simulink model "Standalone_PV_with_MPPT"  (R2024a)
settings: Solver=VariableStepAuto  StartTime=0.0  StopTime=10.0  RelTol=1e-3
libraries: spsSeriesRLCBranchLib x4, spsCurrentMeasurementLib x3, spsMeanLib x2, spsVoltageMeasurementLib x2, spsDiodeLib x1, spsGroundLib x1, spsIGBTLib x1, simulink x1, spsPVArrayLib x1, sps_lib x1
settings Model: Creator=91889  LastModifiedBy=91889

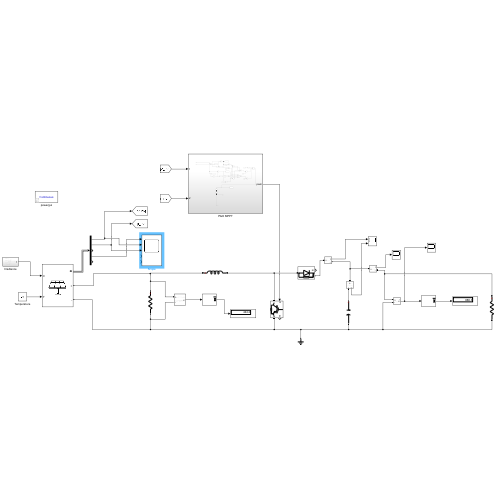
[thumbnail: Simulink's stored preview of the top-level diagram]
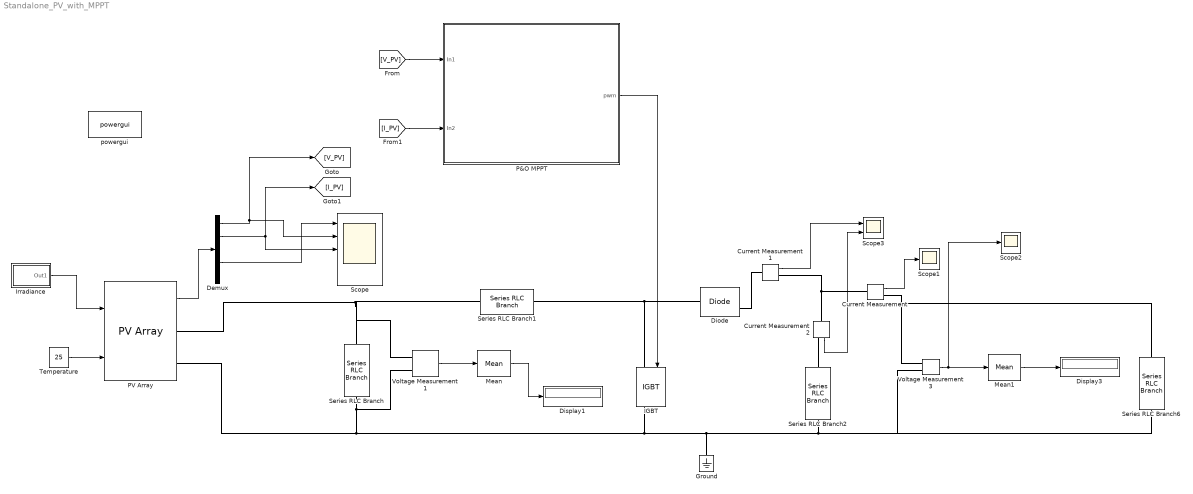
== system Standalone_PV_with_MPPT ==
  Current Measurement : spsCurrentMeasurementLib/Current Measurement  PhasorSimulation=off  OutputType=Complex  PSBequivalent=0
  Current Measurement1 : spsCurrentMeasurementLib/Current Measurement  PhasorSimulation=off  OutputType=Complex  PSBequivalent=0
  Current Measurement2 : spsCurrentMeasurementLib/Current Measurement  PhasorSimulation=off  OutputType=Complex  PSBequivalent=0
  Demux : Demux  Outputs=5
  Diode : spsDiodeLib/Diode  Ron=0.001  Lon=0  Vf=0.8  IC=0  UseSnubber=0  Rs=500  Cs=250e-9  Measurements=on
  Display1 : Display
  Display3 : Display
  Ground : spsGroundLib/Ground  LConnTagsString=a
  IGBT : spsIGBTLib/IGBT  Ron=0.001  Lon=0  Vf=1  Tf=1e-6  Tt=2e-6  IC=0  Rs=1e5  Cs=inf  Measurements=on
  Irradiance : Subsystem
  Mean : spsMeanLib/Mean  Freq=60  Vinit=0  Ts=0
  Mean1 : spsMeanLib/Mean  Freq=60  Vinit=0  Ts=0
  P&O MPPT : Subsystem
  PV Array : spsPVArrayLib/PV Array  Npar=3  Nser=20  PlotType=array @ 1000 W/m2 & specified temperatures  S_vec="[ 1000  500  100 ]"  Temp_C_vec="[ 45 25  ]"  ModuleName=User-defined  PlotWhenSelected=off  Pm=213.15  Ncell=60  Voc=35  Isc=7.84  Vm=29  Im=7.35  beta_Voc_pc=-0.36099  alpha_Isc_pc=0.102  beta_Voc=-0.12635  alpha_Isc=0.0079968  IL=7.8812  I0=2.9282e-10  nI=0.94636  Rsh=184.8932  Rs=0.22133  RobustModel=off  RobustCellTemperature=313.3991  BAL=on  Tc=1e-6  Tfilter=5e-5
  Scope : Scope  NumInputPorts=5
  Scope1 : Scope
  Scope2 : Scope
  Scope3 : Scope  NumInputPorts=2
  Series RLC Branch : spsSeriesRLCBranchLib/Series RLC Branch  LConnTagsString=__new0  RConnTagsString=__new0  BranchType=R  Resistance=100  Inductance=1e-3  SetiL0=off  InitialCurrent=0  Capacitance=1e-6  Setx0=off  InitialVoltage=0  Measurements=None
  Series RLC Branch1 : spsSeriesRLCBranchLib/Series RLC Branch  LConnTagsString=__new0  RConnTagsString=__new0  BranchType=L  Resistance=1  Inductance=5e-3  SetiL0=off  InitialCurrent=0  Capacitance=1e-6  Setx0=off  InitialVoltage=0  Measurements=None
  Series RLC Branch2 : spsSeriesRLCBranchLib/Series RLC Branch  LConnTagsString=__new0  RConnTagsString=__new0  BranchType=C  Resistance=1  Inductance=1e-3  SetiL0=off  InitialCurrent=0  Capacitance=1000e-6  Setx0=off  InitialVoltage=0  Measurements=None
  Series RLC Branch6 : spsSeriesRLCBranchLib/Series RLC Branch  LConnTagsString=__new0  RConnTagsString=__new0  BranchType=R  Resistance=100  Inductance=1e-3  SetiL0=off  InitialCurrent=0  Capacitance=32e-6  Setx0=off  InitialVoltage=0  Measurements=None
  Temperature : Constant  Value=25
  Voltage Measurement1 : spsVoltageMeasurementLib/Voltage Measurement  PhasorSimulation=off  OutputType=Complex  PSBequivalent=0
  Voltage Measurement3 : spsVoltageMeasurementLib/Voltage Measurement  PhasorSimulation=off  OutputType=Complex  PSBequivalent=0
  powergui : sps_lib/powergui  Priority=1  SimulationMode=Continuous  SampleTime=50e-6  frequency=60  Iterations=50  frequencyindice=0  Pbase=100e6  ErrMax=1e-4  UnitsV=kV  UnitsW=MW  buscounter=0  FunctionMessages=off  echomessages=off  EnableUseOfTLC=off  CurrentSourceSwitches=off  DisableSnubberDevices=off  DisableRonSwitches=off  DisableVfSwitches=off  DisplayEquations=off  AutomaticDiscreteSolvers=off  SolverType=Tustin/Backward Euler (TBE)  Interpol=off  ExternalGateDelay=off  methode=off  Ts=100  x0status=blocks  SPID=on  SwTol=0  HookPort=off  NonlinearTolerance=1e-4  nMaxIteration=100  ContinueOnMaxIteration=off  RestoreLinks=warning  ResistiveCurrentMeasurement=off  Frange=[0:2:500]  Ylog=off  Xlog=on  ShowGrid=off  save=off  variable=ZData  structure=0  ZoomFFT=off  StartTime=0.0  cycles=1  DisplayStyle=1  fundamental=60  FreqAxis=off  MaxFrequency=1000  frequencyindicesteady=1  RmsSteady=1  display=off
  wires:
  Irradiance/1(Out1) -> PV Array/1
  Voltage Measurement3/1 -> Mean1/1, Scope2/1
  Mean1/1 -> Display3/1
  PV Array/1 -> Demux/1
  Mean/1 -> Display1/1
  Demux/1 -> Scope/2, [V_PV]
  Current Measurement/1 -> Scope1/1
  Demux/2 -> [I_PV], Scope/3
  Current Measurement2/1 -> Scope3/2
  Current Measurement1/1 -> Scope3/1
  Temperature/1 -> PV Array/2
  [V_PV] -> P&O MPPT/1(In1)
  [I_PV] -> P&O MPPT/2(In2)
  P&O MPPT/1(pwm) -> IGBT/1
  Demux/4 -> Scope/1
  Voltage Measurement1/1 -> Mean/1
  connections:
  Current Measurement2/LConn1 -- Current Measurement1/RConn1 -- Current Measurement/LConn1
  IGBT/LConn1 -- Diode/LConn1 -- Series RLC Branch1/RConn1
  Series RLC Branch6/LConn1 -- Current Measurement/RConn1 -- Voltage Measurement3/LConn1
  IGBT/RConn1 -- Series RLC Branch2/RConn1 -- Series RLC Branch6/RConn1 -- Voltage Measurement3/LConn2 -- Ground/LConn1 -- Voltage Measurement1/LConn2 -- Series RLC Branch/RConn1 -- PV Array/RConn2
  PV Array/RConn1 -- Voltage Measurement1/LConn1 -- Series RLC Branch/LConn1 -- Series RLC Branch1/LConn1
  Current Measurement1/LConn1 -- Diode/RConn1
  Current Measurement2/RConn1 -- Series RLC Branch2/LConn1

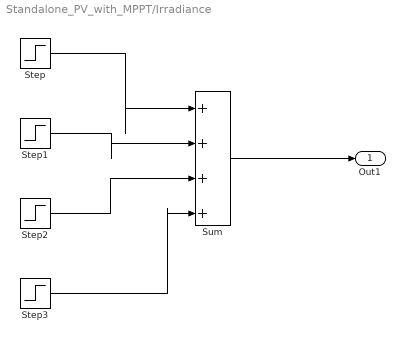
== system Standalone_PV_with_MPPT/Irradiance ==
  Step : Step  Time=0  Before=1200  After=1200  SampleTime=0
  Step1 : Step  Time=3  After=-300  SampleTime=0
  Step2 : Step  Time=5  After=-250  SampleTime=0
  Step3 : Step  Time=8  After=350  SampleTime=0
  Sum : Sum  Inputs=|++++
  Out1 : Outport
  wires:
  Step2/1 -> Sum/3
  Step/1 -> Sum/1
  Sum/1 -> Out1/1
  Step3/1 -> Sum/4
  Step1/1 -> Sum/2

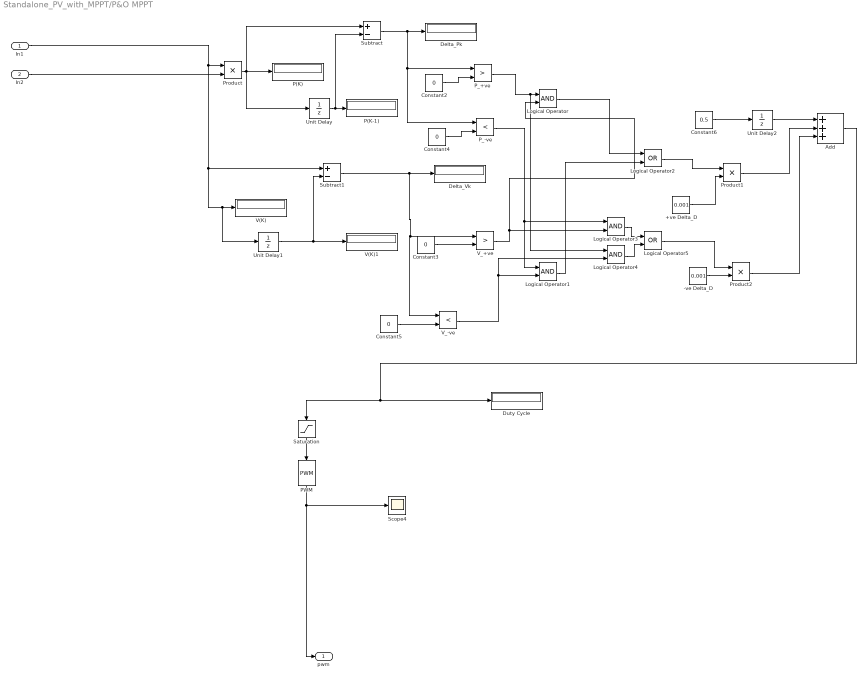
== system Standalone_PV_with_MPPT/P&O MPPT ==
  In1 : Inport
  In2 : Inport  Port=2
  +ve Delta_D : Constant  Value=0.001
  -ve Delta_D : Constant  Value=0.001
  Add : Sum  Inputs=+++
  Constant{2..5} (4 alike) : Constant  Value=0
  Constant6 : Constant  Value=0.5
  Delta_Pk : Display
  Delta_Vk : Display
  Duty Cycle : Display
  Logical Operator{,1,3..4} (4 alike) : Logic  AllPortsSameDT=off  OutDataTypeStr=boolean
  Logical Operator2 : Logic  Operator=OR  AllPortsSameDT=off  OutDataTypeStr=boolean
  Logical Operator5 : Logic  Operator=OR  AllPortsSameDT=off  OutDataTypeStr=boolean
  P(K) : Display
  P(K-1) : Display
  PWM : simulink/Discontinuities/PWM  DisableCoverage=on  Period=50e-6  InitialDelay=0  DisallowZeroDutyCycle=off  RunAtFixedTimeIntervals=off  SampleTime=0.1
  P_+ve : RelationalOperator  Operator=>  OutDataTypeStr=boolean  RndMeth=Simplest  InputSameDT=off
  P_-ve : RelationalOperator  Operator=<  OutDataTypeStr=boolean  RndMeth=Simplest  InputSameDT=off
  Product : Product
  Product1 : Product
  Product2 : Product
  Saturation : Saturate  UpperLimit=0.9  LowerLimit=0.1
  Scope4 : Scope
  Subtract : Sum  Inputs=+-
  Subtract1 : Sum  Inputs=+-
  Unit Delay : UnitDelay  SampleTime=-1  HasFrameUpgradeWarning=on
  Unit Delay1 : UnitDelay  SampleTime=-1  HasFrameUpgradeWarning=on
  Unit Delay2 : UnitDelay  SampleTime=-1  HasFrameUpgradeWarning=on
  V(K) : Display
  V(K)1 : Display
  V_+ve : RelationalOperator  Operator=>  OutDataTypeStr=boolean  RndMeth=Simplest  InputSameDT=off
  V_-ve : RelationalOperator  Operator=<  OutDataTypeStr=boolean  RndMeth=Simplest  InputSameDT=off
  pwm : Outport
  wires:
  PWM/1 -> pwm/1, Scope4/1
  V_+ve/1 -> Logical Operator/2, Logical Operator3/2
  In1/1 -> Subtract1/1, V(K)/1, Unit Delay1/1, Product/1
  Product1/1 -> Add/2
  Unit Delay2/1 -> Add/1
  Subtract/1 -> Delta_Pk/1, P_-ve/1, P_+ve/1
  Logical Operator1/1 -> Logical Operator2/2
  Product2/1 -> Add/3
  Logical Operator/1 -> Logical Operator2/1
  Subtract1/1 -> V_-ve/1, V_+ve/1, Delta_Vk/1
  In2/1 -> Product/2
  Product/1 -> Unit Delay/1, Subtract/1, P(K)/1
  Constant2/1 -> P_+ve/2
  Logical Operator3/1 -> Logical Operator5/1
  P_-ve/1 -> Logical Operator3/1, Logical Operator1/1
  Logical Operator5/1 -> Product2/1
  V_-ve/1 -> Logical Operator4/2, Logical Operator1/2
  -ve Delta_D/1 -> Product2/2
  Constant5/1 -> V_-ve/2
  +ve Delta_D/1 -> Product1/2
  Logical Operator2/1 -> Product1/1
  Unit Delay/1 -> Subtract/2, P(K-1)/1
  Add/1 -> Duty Cycle/1, Saturation/1
  P_+ve/1 -> Logical Operator4/1, Logical Operator/1
  Unit Delay1/1 -> Subtract1/2, V(K)1/1
  Constant6/1 -> Unit Delay2/1
  Saturation/1 -> PWM/1
  Constant4/1 -> P_-ve/2
  Logical Operator4/1 -> Logical Operator5/2
  Constant3/1 -> V_+ve/2
